simulink model "quadcopter_control_2018a"  (R2018a)
settings: Solver=VariableStepAuto  StartTime=0.0  StopTime=totTime  RelTol=1e-3
values from neighbouring files (symbols this model uses):
  armLength = 0.1    [quadcopter.m]    (also in quadcopter_control_RL.m)
  dragFactor = 0.1    [quadcopter.m]    (also in quadcopter_control_RL.m)
  iX = 0.03    [quadcopter.m]    (also in quadcopter_control_RL.m)
  iY = 0.03    [quadcopter.m]    (also in quadcopter_control_RL.m)
  iZ = 0.03    [quadcopter.m]    (also in quadcopter_control_RL.m)
  mass = 0.25    [quadcopter.m]    (also in quadcopter_control_RL.m)
  phi0 = 0.0    (= 0)    [quadcopter.m]    (also in quadcopter_control_RL.m = omega_vec_next(1))
  phiDot0 = 0.0    (= 0)    [quadcopter.m]    (also in quadcopter_control_RL.m = omega_vec_next(4))
  psi0 = 0.0    (= 0)    [quadcopter.m]    (also in quadcopter_control_RL.m = omega_vec_next(3))
  psiDot0 = 0.0    (= 0)    [quadcopter.m]    (also in quadcopter_control_RL.m = omega_vec_next(6))
  theta0 = 0.0    (= 0)    [quadcopter.m]    (also in quadcopter_control_RL.m = omega_vec_next(2))
  thetaDot0 = 0.0    (= 0)    [quadcopter.m]    (also in quadcopter_control_RL.m = omega_vec_next(5))
  thrustFactor = 0.1    [quadcopter.m]    (also in quadcopter_control_RL.m)
  trajectory = zeros(length(t),4)    [quadcopter.m]
  Ts = 0.1    [quadcopter.m]
  x0 = 0.0    (= 0)    [quadcopter.m]    (also in quadcopter_control_RL.m = x_vec_next(1))
  xDot0 = 0.0    (= 0)    [quadcopter.m]    (also in quadcopter_control_RL.m = x_vec_next(4))
  y0 = 0.0    (= 0)    [quadcopter.m]    (also in quadcopter_control_RL.m = x_vec_next(2))
  yDot0 = 0.0    (= 0)    [quadcopter.m]    (also in quadcopter_control_RL.m = x_vec_next(5))
  z0 = 0.00000001    (= 1e-08)    [quadcopter.m]    (also in quadcopter_control_RL.m = x_vec_next(3))
  zDot0 = 0.00000001    (= 1e-08)    [quadcopter.m]    (also in quadcopter_control_RL.m = x_vec_next(6))
libraries: simulink x1
settings Model: Creator=Ramprasad  LastModifiedBy=vickneshbalabaskara
settings DebuggingCC: LibraryContextMissingDiagnostic=warning
settings SFSimCC: SimUseLocalCustomCode=on
settings RTWCC: RTWUseLocalCustomCode=on

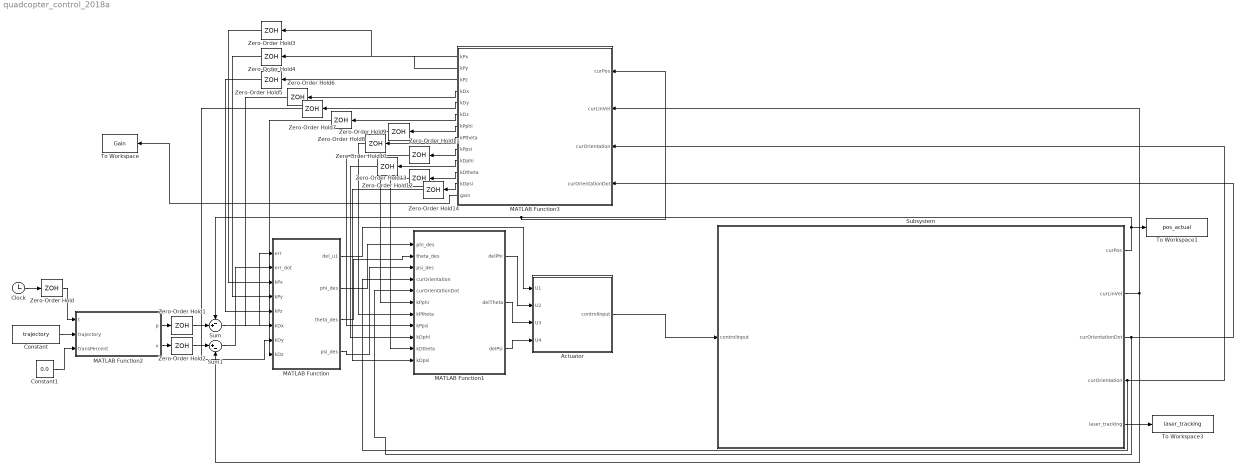
== system quadcopter_control_2018a ==
  Actuator : Subsystem
  Clock : Clock
  Constant : Constant  Value=trajectory
  Constant1 : Constant  Value=0.0
  MATLAB Function : MATLAB Function  TreatAsAtomicUnit=on
  MATLAB Function1 : MATLAB Function  TreatAsAtomicUnit=on
  MATLAB Function2 : MATLAB Function  TreatAsAtomicUnit=on
  MATLAB Function3 : MATLAB Function  TreatAsAtomicUnit=on
  Subsystem : Subsystem
  Sum : Sum  Inputs=-+|
  Sum1 : Sum  Inputs=|+-
  To Workspace : ToWorkspace  VariableName=Gain  SaveFormat=Timeseries  SampleTime=Ts
  To Workspace1 : ToWorkspace  VariableName=pos_actual  SaveFormat=Structure With Time  SampleTime=-1
  To Workspace3 : ToWorkspace  VariableName=laser_tracking  SaveFormat=Structure With Time  SampleTime=-1
  Zero-Order Hold{,1..14} (15 alike) : ZeroOrderHold  SampleTime=0.001
  wires:
  Actuator/1(controlInput) -> Subsystem/1(controlInput)
  Constant/1 -> MATLAB Function2/2(trajectory)
  Clock/1 -> Zero-Order Hold/1
  Zero-Order Hold/1 -> MATLAB Function2/1(t)
  MATLAB Function/2(phi_des) -> MATLAB Function1/1(phi_des)
  MATLAB Function/3(theta_des) -> MATLAB Function1/2(theta_des)
  MATLAB Function/4(psi_des) -> MATLAB Function1/3(psi_des)
  MATLAB Function2/1(p) -> Zero-Order Hold1/1
  MATLAB Function2/2(v) -> Zero-Order Hold2/1
  Zero-Order Hold1/1 -> Sum/2
  Zero-Order Hold2/1 -> Sum1/1
  Sum/1 -> MATLAB Function/1(err)
  Sum1/1 -> MATLAB Function/2(err_dot)
  Subsystem/1(curPos) -> MATLAB Function3/1(curPos), Sum/1, To Workspace1/1
  Constant1/1 -> MATLAB Function2/3(transPercent)
  MATLAB Function/1(del_u1) -> Actuator/1(U1)
  MATLAB Function1/1(delPhi) -> Actuator/2(U2)
  MATLAB Function1/2(delTheta) -> Actuator/3(U3)
  MATLAB Function1/3(delPsi) -> Actuator/4(U4)
  Subsystem/5(laser_tracking) -> To Workspace3/1
  Subsystem/2(curLinVel) -> Sum1/2, MATLAB Function3/2(curLinVel)
  Subsystem/4(curOrientation) -> MATLAB Function1/4(curOrientation), MATLAB Function3/3(curOrientation)
  Subsystem/3(curOrientationDot) -> MATLAB Function1/5(curOrientationDot), MATLAB Function3/4(curOrientationDot)
  MATLAB Function3/1(kPx) -> Zero-Order Hold3/1
  MATLAB Function3/2(kPy) -> Zero-Order Hold4/1
  MATLAB Function3/3(kPz) -> Zero-Order Hold5/1
  MATLAB Function3/4(kDx) -> Zero-Order Hold6/1
  MATLAB Function3/5(kDy) -> Zero-Order Hold7/1
  MATLAB Function3/6(kDz) -> Zero-Order Hold8/1
  MATLAB Function3/7(kPphi) -> Zero-Order Hold9/1
  MATLAB Function3/8(kPtheta) -> Zero-Order Hold10/1
  MATLAB Function3/9(kPpsi) -> Zero-Order Hold11/1
  MATLAB Function3/10(kDphi) -> Zero-Order Hold12/1
  MATLAB Function3/11(kDtheta) -> Zero-Order Hold13/1
  MATLAB Function3/12(kDpsi) -> Zero-Order Hold14/1
  Zero-Order Hold3/1 -> MATLAB Function/3(kPx)
  Zero-Order Hold4/1 -> MATLAB Function/4(kPy)
  Zero-Order Hold5/1 -> MATLAB Function/5(kPz)
  Zero-Order Hold6/1 -> MATLAB Function/6(kDx)
  Zero-Order Hold7/1 -> MATLAB Function/7(kDy)
  Zero-Order Hold8/1 -> MATLAB Function/8(kDz)
  Zero-Order Hold9/1 -> MATLAB Function1/6(kPphi)
  Zero-Order Hold10/1 -> MATLAB Function1/7(kPtheta)
  Zero-Order Hold11/1 -> MATLAB Function1/8(kPpsi)
  Zero-Order Hold12/1 -> MATLAB Function1/9(kDphi)
  Zero-Order Hold13/1 -> MATLAB Function1/10(kDtheta)
  Zero-Order Hold14/1 -> MATLAB Function1/11(kDpsi)
  MATLAB Function3/13(gain) -> To Workspace/1

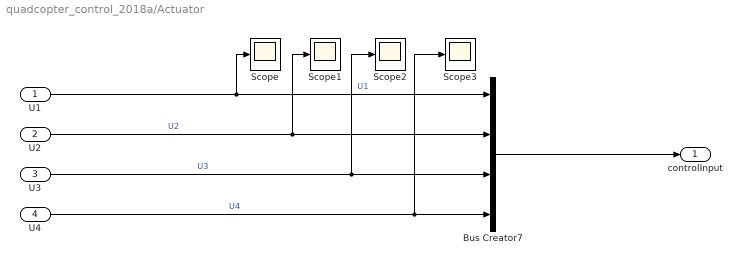
== system quadcopter_control_2018a/Actuator ==
  U1 : Inport
  U2 : Inport  Port=2
  U3 : Inport  Port=3
  U4 : Inport  Port=4
  Bus Creator7 : BusCreator  Inputs=4
  Scope{,1..3} (4 alike) : Scope
  controlInput : Outport
  wires:
  U1/1 -> Scope/1, Bus Creator7/1  "U1"
  U4/1 -> Scope3/1, Bus Creator7/4  "U4"
  Bus Creator7/1 -> controlInput/1
  U2/1 -> Scope1/1, Bus Creator7/2  "U2"
  U3/1 -> Scope2/1, Bus Creator7/3  "U3"

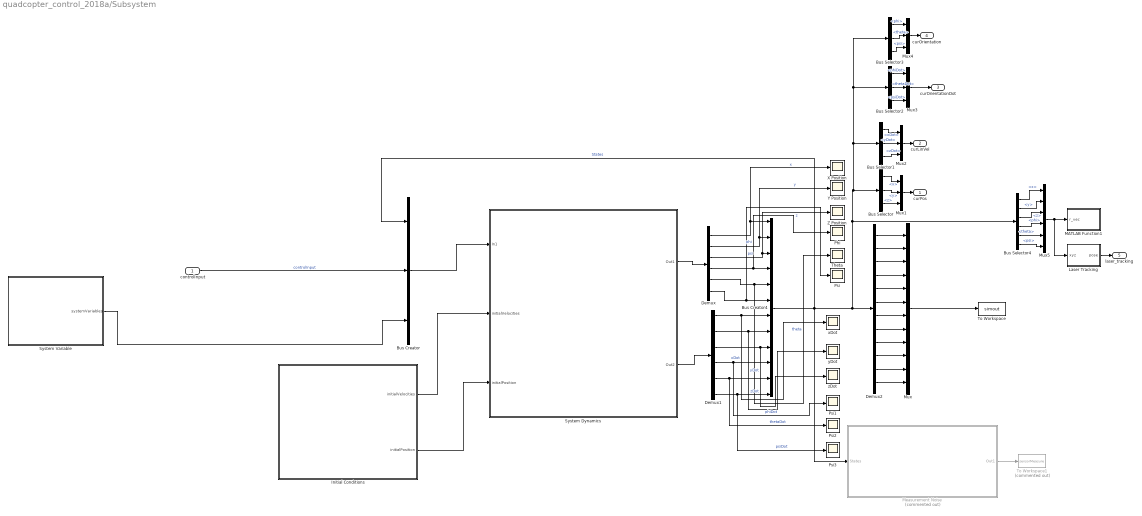
== system quadcopter_control_2018a/Subsystem ==
  controlInput : Inport
  Bus Creator : BusCreator  Inputs=3
  Bus Creator4 : BusCreator  Inputs=12
  Bus Selector : BusSelector  OutputSignals=x,y,z
  Bus Selector1 : BusSelector  OutputSignals=xDot,yDot,zDot
  Bus Selector2 : BusSelector  OutputSignals=phiDot,thetaDot,psiDot
  Bus Selector3 : BusSelector  OutputSignals=phi,theta,psi
  Bus Selector4 : BusSelector  OutputSignals=x,y,z,phi,theta,psi
  Demux : Demux  Outputs=6
  Demux1 : Demux  Outputs=6
  Demux2 : Demux  Outputs=12
  Initial Conditions : Subsystem
  Laser Tracking : MATLAB Function  TreatAsAtomicUnit=on
  MATLAB Function1 : MATLAB Function  TreatAsAtomicUnit=on
  Measurement Noise : Subsystem  Commented=on
  Mux : Mux  Inputs=12
  Mux{1..4} (4 alike) : Mux  Inputs=3
  Mux5 : Mux  Inputs=6
  Phi : Scope
  Psi{,1..3} (4 alike) : Scope
  System Dynamics : Subsystem
  System Variable : Subsystem
  Theta : Scope
  To Workspace : ToWorkspace  VariableName=simout  SaveFormat=Timeseries  SampleTime=Ts
  To Workspace1 : ToWorkspace  Commented=on  VariableName=sensorMeasure  SaveFormat=Timeseries  SampleTime=-1
  X Position : Scope
  Y Position : Scope
  Z Position : Scope
  xDot : Scope
  yDot : Scope
  zDot : Scope
  curPos : Outport
  curLinVel : Outport  Port=2
  curOrientationDot : Outport  Port=3
  curOrientation : Outport  Port=4
  laser_tracking : Outport  Port=5
  wires:
  Demux1/1 -> xDot/1, Bus Creator4/7  "xDot"
  Demux2/6 -> Mux/6
  Demux/6 -> Psi/1, Bus Creator4/6  "psi"
  Demux1/2 -> yDot/1, Bus Creator4/8  "yDot"
  Mux/1 -> To Workspace/1
  Demux2/9 -> Mux/9
  Demux1/6 -> Psi3/1, Bus Creator4/12  "psiDot"
  Measurement Noise/1(Out1) -> To Workspace1/1
  Demux/4 -> Phi/1, Bus Creator4/4  "phi"
  System Dynamics/1(Out1) -> Demux/1
  Initial Conditions/1(initialVelocities) -> System Dynamics/2(initialVelocities)
  Initial Conditions/2(initialPosition) -> System Dynamics/3(initialPosition)
  Bus Creator/1 -> System Dynamics/1(In1)
  Demux/2 -> Bus Creator4/2, Y Position/1  "y"
  Demux2/5 -> Mux/5
  System Dynamics/2(Out2) -> Demux1/1
  Demux2/3 -> Mux/3
  Demux/1 -> Bus Creator4/1, X Position/1  "x"
  Demux2/8 -> Mux/8
  Demux2/7 -> Mux/7
  Demux2/2 -> Mux/2
  Demux2/12 -> Mux/12
  Demux1/4 -> Psi1/1, Bus Creator4/10  "phiDot"
  Demux/5 -> Theta/1, Bus Creator4/5  "theta"
  Demux/3 -> Z Position/1, Bus Creator4/3  "z"
  Demux2/1 -> Mux/1
  Demux2/10 -> Mux/10
  Bus Creator4/1 -> Bus Creator/1, Bus Selector3/1, Bus Selector2/1, Bus Selector1/1, Bus Selector/1, Bus Selector4/1, Demux2/1, Measurement Noise/1(States)  "States"
  Demux2/11 -> Mux/11
  Demux1/5 -> Psi2/1, Bus Creator4/11  "thetaDot"
  Demux2/4 -> Mux/4
  Demux1/3 -> zDot/1, Bus Creator4/9  "zDot"
  System Variable/1(systemVariables) -> Bus Creator/3
  Bus Selector/3 -> Mux1/3  "<z>"
  Bus Selector/2 -> Mux1/2  "<y>"
  Bus Selector/1 -> Mux1/1  "<x>"
  Mux1/1 -> curPos/1
  Bus Selector1/2 -> Mux2/2  "<yDot>"
  Bus Selector1/3 -> Mux2/3  "<zDot>"
  Bus Selector1/1 -> Mux2/1  "<xDot>"
  Mux2/1 -> curLinVel/1
  Bus Selector3/1 -> Mux4/1  "<phi>"
  Bus Selector3/2 -> Mux4/2  "<theta>"
  Bus Selector3/3 -> Mux4/3  "<psi>"
  Mux4/1 -> curOrientation/1
  Bus Selector2/1 -> Mux3/1  "<phiDot>"
  Bus Selector2/2 -> Mux3/2  "<thetaDot>"
  Mux3/1 -> curOrientationDot/1
  Bus Selector2/3 -> Mux3/3  "<psiDot>"
  Bus Selector4/1 -> Mux5/1  "<x>"
  Bus Selector4/2 -> Mux5/2  "<y>"
  Bus Selector4/3 -> Mux5/3  "<z>"
  Bus Selector4/4 -> Mux5/4  "<phi>"
  Bus Selector4/5 -> Mux5/5  "<theta>"
  Bus Selector4/6 -> Mux5/6  "<psi>"
  Mux5/1 -> Laser Tracking/1(xyz), MATLAB Function1/1(r_vec)
  controlInput/1 -> Bus Creator/2  "controlInput"
  Laser Tracking/1(pose) -> laser_tracking/1

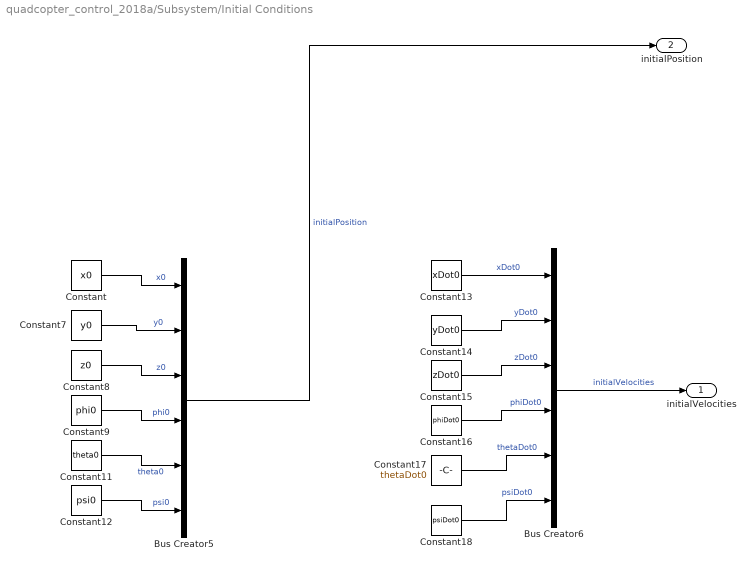
== system quadcopter_control_2018a/Subsystem/Initial Conditions ==
  Bus Creator5 : BusCreator  Inputs=6
  Bus Creator6 : BusCreator  Inputs=6
  Constant : Constant  Value=x0
  Constant11 : Constant  Value=theta0
  Constant12 : Constant  Value=psi0
  Constant13 : Constant  Value=xDot0
  Constant14 : Constant  Value=yDot0
  Constant15 : Constant  Value=zDot0
  Constant16 : Constant  Value=phiDot0
  Constant17 : Constant  Value=thetaDot0
  Constant18 : Constant  Value=psiDot0
  Constant7 : Constant  Value=y0
  Constant8 : Constant  Value=z0
  Constant9 : Constant  Value=phi0
  initialVelocities : Outport
  initialPosition : Outport  Port=2
  wires:
  Constant9/1 -> Bus Creator5/4  "phi0"
  Constant14/1 -> Bus Creator6/2  "yDot0"
  Constant17/1 -> Bus Creator6/5  "thetaDot0"
  Constant18/1 -> Bus Creator6/6  "psiDot0"
  Constant13/1 -> Bus Creator6/1  "xDot0"
  Constant11/1 -> Bus Creator5/5  "theta0"
  Constant8/1 -> Bus Creator5/3  "z0"
  Constant16/1 -> Bus Creator6/4  "phiDot0"
  Constant12/1 -> Bus Creator5/6  "psi0"
  Constant15/1 -> Bus Creator6/3  "zDot0"
  Constant/1 -> Bus Creator5/1  "x0"
  Bus Creator6/1 -> initialVelocities/1  "initialVelocities"
  Constant7/1 -> Bus Creator5/2  "y0"
  Bus Creator5/1 -> initialPosition/1  "initialPosition"

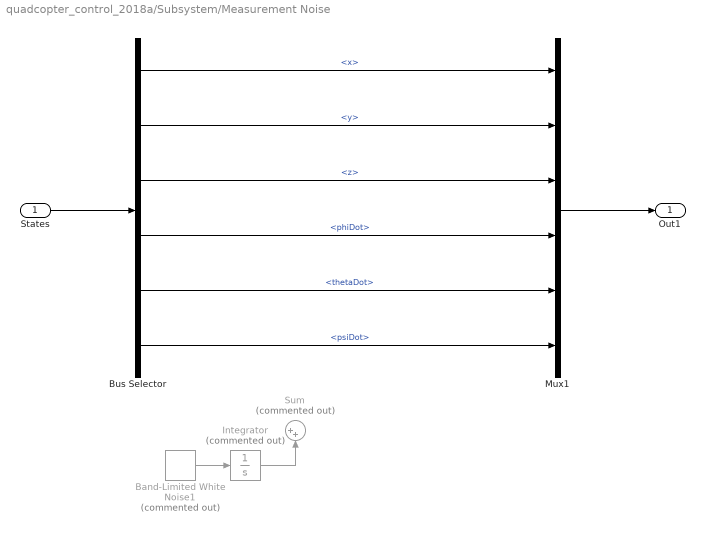
== system quadcopter_control_2018a/Subsystem/Measurement Noise ==
  States : Inport
  Band-Limited White Noise1 : simulink/Sources/Band-Limited White Noise  Commented=on  Cov=[0.0]  Ts=Ts  seed=[23341]
  Bus Selector : BusSelector  OutputSignals=x,y,z,phiDot,thetaDot,psiDot
  Integrator : Integrator  Commented=on
  Mux1 : Mux  Inputs=6
  Sum : Sum  Commented=on  Inputs=|++
  Out1 : Outport
  wires:
  Integrator/1 -> Sum/2
  Bus Selector/3 -> Mux1/3  "<z>"
  Bus Selector/2 -> Mux1/2  "<y>"
  Mux1/1 -> Out1/1
  Band-Limited White Noise1/1 -> Integrator/1
  Bus Selector/4 -> Mux1/4  "<phiDot>"
  States/1 -> Bus Selector/1
  Bus Selector/6 -> Mux1/6  "<psiDot>"
  Bus Selector/5 -> Mux1/5  "<thetaDot>"
  Bus Selector/1 -> Mux1/1  "<x>"

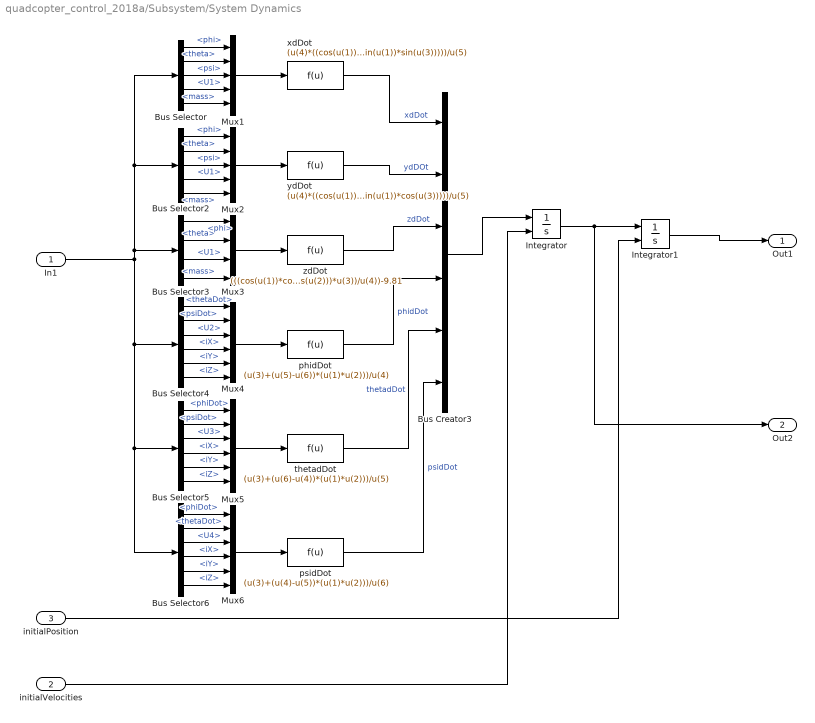
== system quadcopter_control_2018a/Subsystem/System Dynamics ==
  In1 : Inport
  initialVelocities : Inport  Port=2
  initialPosition : Inport  Port=3
  Bus Creator3 : BusCreator  Inputs=6
  Bus Selector : BusSelector  OutputSignals=States.phi,States.theta,States.psi,controlInput.U1,systemVariables.mass
  Bus Selector2 : BusSelector  OutputSignals=States.phi,States.theta,States.psi,controlInput.U1,systemVariables.mass
  Bus Selector3 : BusSelector  OutputSignals=States.phi,States.theta,controlInput.U1,systemVariables.mass
  Bus Selector4 : BusSelector  OutputSignals=States.thetaDot,States.psiDot,controlInput.U2,systemVariables.iX,systemVariables.iY,systemVariables.iZ
  Bus Selector5 : BusSelector  OutputSignals=States.phiDot,States.psiDot,controlInput.U3,systemVariables.iX,systemVariables.iY,systemVariables.iZ
  Bus Selector6 : BusSelector  OutputSignals=States.phiDot,States.thetaDot,controlInput.U4,systemVariables.iX,systemVariables.iY,systemVariables.iZ
  Integrator : Integrator  InitialConditionSource=external
  Integrator1 : Integrator  InitialConditionSource=external
  Mux1 : Mux  Inputs=5
  Mux2 : Mux  Inputs=5
  Mux3 : Mux
  Mux4 : Mux  Inputs=6
  Mux5 : Mux  Inputs=6
  Mux6 : Mux  Inputs=6
  phidDot : Fcn  Expr=(u(3)+(u(5)-u(6))*(u(1)*u(2)))/u(4)
  psidDot : Fcn  Expr=(u(3)+(u(4)-u(5))*(u(1)*u(2)))/u(6)
  thetadDot : Fcn  Expr=(u(3)+(u(6)-u(4))*(u(1)*u(2)))/u(5)
  xdDot : Fcn  Expr=(u(4)*((cos(u(1))*sin(u(2))*cos(u(3)))+(sin(u(1))*sin(u(3)))))/u(5)
  ydDot : Fcn  Expr=(u(4)*((cos(u(1))*sin(u(2))*sin(u(3)))-(sin(u(1))*cos(u(3)))))/u(5)
  zdDot : Fcn  Expr=(((cos(u(1))*cos(u(2)))*u(3))/u(4))-9.81
  Out1 : Outport
  Out2 : Outport  Port=2
  wires:
  initialPosition/1 -> Integrator1/2
  xdDot/1 -> Bus Creator3/1  "xdDot"
  Bus Selector2/2 -> Mux2/2  "<theta>"
  Bus Selector4/5 -> Mux4/5  "<iY>"
  Bus Selector2/4 -> Mux2/4  "<U1>"
  Bus Selector4/3 -> Mux4/3  "<U2>"
  thetadDot/1 -> Bus Creator3/5  "thetadDot"
  Bus Selector5/2 -> Mux5/2  "<psiDot>"
  Bus Selector2/1 -> Mux2/1  "<phi>"
  Mux5/1 -> thetadDot/1
  Bus Selector6/4 -> Mux6/4  "<iX>"
  Bus Selector5/6 -> Mux5/6  "<iZ>"
  Bus Selector6/2 -> Mux6/2  "<thetaDot>"
  phidDot/1 -> Bus Creator3/4  "phidDot"
  Bus Selector2/3 -> Mux2/3  "<psi>"
  In1/1 -> Bus Selector4/1, Bus Selector5/1, Bus Selector6/1, Bus Selector3/1, Bus Selector2/1, Bus Selector/1
  Bus Selector5/3 -> Mux5/3  "<U3>"
  Bus Selector3/2 -> Mux3/2  "<theta>"
  Bus Selector3/1 -> Mux3/1  "<phi>"
  initialVelocities/1 -> Integrator/2
  Bus Selector/3 -> Mux1/3  "<psi>"
  Mux6/1 -> psidDot/1
  Bus Selector5/4 -> Mux5/4  "<iX>"
  Bus Selector/4 -> Mux1/4  "<U1>"
  Bus Selector/1 -> Mux1/1  "<phi>"
  Mux4/1 -> phidDot/1
  Bus Selector4/6 -> Mux4/6  "<iZ>"
  Bus Selector2/5 -> Mux2/5  "<mass>"
  Bus Creator3/1 -> Integrator/1
  Bus Selector6/6 -> Mux6/6  "<iZ>"
  Bus Selector3/3 -> Mux3/3  "<U1>"
  Mux2/1 -> ydDot/1
  Bus Selector6/3 -> Mux6/3  "<U4>"
  Bus Selector6/1 -> Mux6/1  "<phiDot>"
  zdDot/1 -> Bus Creator3/3  "zdDot"
  Bus Selector5/1 -> Mux5/1  "<phiDot>"
  Bus Selector4/2 -> Mux4/2  "<psiDot>"
  Bus Selector6/5 -> Mux6/5  "<iY>"
  Bus Selector4/4 -> Mux4/4  "<iX>"
  Bus Selector4/1 -> Mux4/1  "<thetaDot>"
  Mux3/1 -> zdDot/1
  Integrator/1 -> Integrator1/1, Out2/1
  psidDot/1 -> Bus Creator3/6  "psidDot"
  Integrator1/1 -> Out1/1
  Bus Selector/5 -> Mux1/5  "<mass>"
  ydDot/1 -> Bus Creator3/2  "ydDOt"
  Bus Selector5/5 -> Mux5/5  "<iY>"
  Bus Selector/2 -> Mux1/2  "<theta>"
  Bus Selector3/4 -> Mux3/4  "<mass>"
  Mux1/1 -> xdDot/1

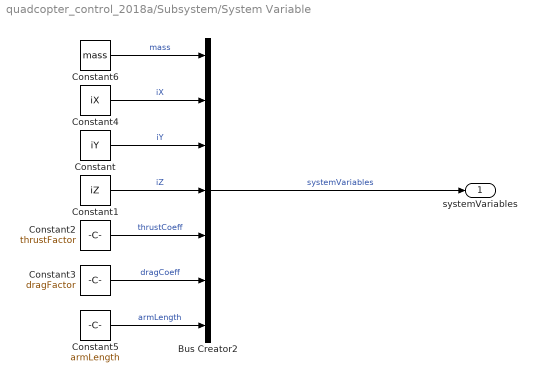
== system quadcopter_control_2018a/Subsystem/System Variable ==
  Bus Creator2 : BusCreator  Inputs=7
  Constant : Constant  Value=iY
  Constant1 : Constant  Value=iZ
  Constant2 : Constant  Value=thrustFactor
  Constant3 : Constant  Value=dragFactor
  Constant4 : Constant  Value=iX
  Constant5 : Constant  Value=armLength
  Constant6 : Constant  Value=mass
  systemVariables : Outport
  wires:
  Constant6/1 -> Bus Creator2/1  "mass"
  Constant2/1 -> Bus Creator2/5  "thrustCoeff"
  Constant/1 -> Bus Creator2/3  "iY"
  Constant1/1 -> Bus Creator2/4  "iZ"
  Constant3/1 -> Bus Creator2/6  "dragCoeff"
  Constant4/1 -> Bus Creator2/2  "iX"
  Constant5/1 -> Bus Creator2/7  "armLength"
  Bus Creator2/1 -> systemVariables/1  "systemVariables"

== matlab function quadcopter_control_2018a/Subsystem/MATLAB Function1 ==
  settings: updateMethod=DISCRETE
  data: r_vec input
function drawDrone(r_vec)
%#codegen
coder.extrinsic('evalin');
coder.extrinsic('load');
coder.extrinsic('animatedline');
% persistent figNum axisHandel Sim_Exact points3D;

% if isempty(Sim_Exact)
%     Sim_Exact = evalin('base','Sim_Exact');
%     a.points3D = zeros(21,3,'double');
%     a = load('points3D.mat');
%     points3D = zeros(21,3,'double');
%     points3D = a.points3D;
% end

x = r_vec(1);
y = r_vec(2);
z = r_vec(3);
phi = r_vec(4);
theta = r_vec(5);
psi = r_vec(6);

T06 = [cos(psi)*cos(theta) (cos(psi)*sin(theta)*sin(phi))-(sin(psi)*cos(phi)) (cos(phi)*sin(theta)*cos(psi))+(sin(phi)*sin(psi)) x;...
       sin(psi)*cos(theta) (sin(phi)*sin(theta)*sin(psi))+(cos(phi)*cos(psi)) (sin(psi)*sin(theta)*cos(phi))-(cos(psi)*sin(phi)) y;...
       -sin(theta) (cos(theta)*sin(phi)) (cos(theta)*cos(phi)) z;...
       0 0 0 1];

R06 = T06(1:3,1:3);

% P1 =[ 0
%     0
%     0.29];
% P2 = [ 0.27*cos(x)*cos(y);
%     0.27*cos(y)*sin(x);
%     0.29 - 0.27*sin(y)];
% P3 = [ 0.27*cos(x)*cos(y) - 0.07*cos(x)*sin(y)*sin(z) + 0.07*cos(x)*cos(y)*cos(z);
%     0.27*cos(y)*sin(x) - 0.07*sin(x)*sin(y)*sin(z) + 0.07*cos(y)*cos(z)*sin(x);
%     0.29 - 0.07*cos(y)*sin(z) - 0.07*cos(z)*sin(y) - 0.27*sin(y)];
% 
% P4 = [ 0.27*cos(x)*cos(y) - 0.07*cos(x)*sin(y)*sin(z) + 0.07*cos(x)*cos(y)*cos(z) - 0.302*cos(x)*cos(y)*sin(z) - 0.302*cos(x)*cos(z)*sin(y);
%     0.27*cos(y)*sin(x) - 0.302*cos(y)*sin(x)*sin(z) - 0.302*cos(z)*sin(x)*sin(y) - 0.07*sin(x)*sin(y)*sin(z) + 0.07*cos(y)*cos(z)*sin(x);
%     0.302*sin(y)*sin(z) - 0.302*cos(y)*cos(z) - 0.07*cos(y)*sin(z) - 0.07*cos(z)*sin(y) - 0.27*sin(y) + 0.29];
% P5 = [ 0.27*cos(x)*cos(y) - 0.07*cos(x)*sin(y)*sin(z) + 0.07*cos(x)*cos(y)*cos(z) - 0.302*cos(x)*cos(y)*sin(z) - 0.302*cos(x)*cos(z)*sin(y)
%     0.27*cos(y)*sin(x) - 0.302*cos(y)*sin(x)*sin(z) - 0.302*cos(z)*sin(x)*sin(y) - 0.07*sin(x)*sin(y)*sin(z) + 0.07*cos(y)*cos(z)*sin(x)
%     0.302*sin(y)*sin(z) - 0.302*cos(y)*cos(z) - 0.07*cos(y)*sin(z) - 0.07*cos(z)*sin(y) - 0.27*sin(y) + 0.29];
% 
% P6 =[ 0.27*cos(x)*cos(y) - 0.07*cos(x)*sin(y)*sin(z) - 0.072*sin(x)*sin(phi)*sin(theta) + 0.07*cos(x)*cos(y)*cos(z) - 0.302*cos(x)*cos(y)*sin(z) - 0.302*cos(x)*cos(z)*sin(y) - 0.072*cos(x)*cos(y)*cos(theta)*sin(z) - 0.072*cos(x)*cos(z)*cos(theta)*sin(y) - 0.072*cos(x)*cos(y)*cos(z)*cos(phi)*sin(theta) + 0.072*cos(x)*cos(phi)*sin(y)*sin(z)*sin(theta);
%     0.27*cos(y)*sin(x) - 0.302*cos(y)*sin(x)*sin(z) - 0.302*cos(z)*sin(x)*sin(y) + 0.072*cos(x)*sin(phi)*sin(theta) - 0.07*sin(x)*sin(y)*sin(z) + 0.07*cos(y)*cos(z)*sin(x) - 0.072*cos(y)*cos(theta)*sin(x)*sin(z) - 0.072*cos(z)*cos(theta)*sin(x)*sin(y) - 0.072*cos(y)*cos(z)*cos(phi)*sin(x)*sin(theta) + 0.072*cos(phi)*sin(x)*sin(y)*sin(z)*sin(theta);
%     0.302*sin(y)*sin(z) - 0.302*cos(y)*cos(z) - 0.07*cos(y)*sin(z) - 0.07*cos(z)*sin(y) - 0.27*sin(y) + 0.072*cos(theta)*sin(y)*sin(z) - 0.072*cos(y)*cos(z)*cos(theta) + 0.072*cos(y)*cos(phi)*sin(z)*sin(theta) + 0.072*cos(z)*cos(phi)*sin(y)*sin(theta) + 0.29];

Q1 = [(0.1/sqrt(2));(0.1/sqrt(2));0];
Q2 = [-(0.1/sqrt(2));(0.1/sqrt(2));0];
Q3 = [(0.1/sqrt(2));-(0.1/sqrt(2));0];
Q4 = [-(0.1/sqrt(2));-(0.1/sqrt(2));0];

R1 = R06*Q1;
R2 = R06*Q2;
R3 = R06*Q3;
R4 = R06*Q4;

P1 = [x+R1(1);y+R1(2);z+R1(3)];
P2 = [x+R2(1);y+R2(2);z+R2(3)];
P3 = [x+R3(1);y+R3(2);z+R3(3)];
P4 = [x+R4(1);y+R4(2);z+R4(3)];

% if isempty(figNum)
%     figNum = figure(1);
%     hold on;
%     plot3([0;P1(1);P2(1);P3(1);P4(1);P5(1);P6(1)],...
%         [0;P1(2);P2(2);P3(2);P4(2);P5(2);P6(2)],...
%         [0;P1(3);P2(3);P3(3);P4(3);P5(3);P6(3)],'k','linewidth',2);
%     axisHandel = gca;
%     plot3([P6(1);P6(1)+T06(1,1)*.1],...
%         [P6(2);P6(2)+T06(2,1)*.1],...
%         [P6(3);P6(3)+T06(3,1)*.1],'r','Parent',axisHandel);
%     plot3([P6(1);P6(1)+T06(1,2)*.1],...
%         [P6(2);P6(2)+T06(2,2)*.1],...
%         [P6(3);P6(3)+T06(3,2)*.1],'g','Parent',axisHandel);
%     plot3([P6(1);P6(1)+T06(1,3)*.1],...
%         [P6(2);P6(2)+T06(2,3)*.1],...
%         [P6(3);P6(3)+T06(3,3)*.1],'b','Parent',axisHandel);
%     plot3(points3D(:,1),points3D(:,2),points3D(:,3),'m','Parent',axisHandel);
%     hold off;
%     axis([-.75 .75 -.75 .75 -.4 .75]);
%     axisHandel = gca;
% else
figure(1)
plot3([x;P1(1)],[y;P1(2)],[z;P1(3)],'k','linewidth',2,'Parent',gca);
hold on;
plot3([x;P2(1)],[y;P2(2)],[z;P2(3)],'k','linewidth',2,'Parent',gca);
hold on;
plot3([x;P3(1)],[y;P3(2)],[z;P3(3)],'k','linewidth',2,'Parent',gca);
hold on;
plot3([x;P4(1)],[y;P4(2)],[z;P4(3)],'k','linewidth',2,'Parent',gca);
hold on;
plot3([x;x+T06(1,1)*.1],[y;y+T06(2,1)*.1],[z;z+T06(3,1)*.1],'r','Parent',gca);
plot3([x;x+T06(1,2)*.1],[y;y+T06(2,2)*.1],[z;z+T06(3,2)*.1],'g','Parent',gca);
plot3([x;x+T06(1,3)*.1],[y;y+T06(2,3)*.1],[z;z+T06(3,3)*.1],'b','Parent',gca);
% plot3([P6(1);P6(1)+T06(1,2)*.1],...
%     [P6(2);P6(2)+T06(2,2)*.1],...
%     [P6(3);P6(3)+T06(3,2)*.1],'g','Parent',gca);
% plot3([P6(1);P6(1)+T06(1,3)*.1],...
%     [P6(2);P6(2)+T06(2,3)*.1],...
%     [P6(3);P6(3)+T06(3,3)*.1],'b','Parent',gca);
% plot3(x,y,z,'m','Parent',gca);
hold off;
axis([-0.1 1.1 -0.1 1.1 0.0 1.1]);
end

== matlab function quadcopter_control_2018a/MATLAB Function2 ==
  data: t input; p output; trajectory input; transPercent input; v output
function [p,v] = constAccelInterp(t,trajectory,transPercent)
pTime = trajectory(:,1);
[n,m] = size(trajectory);
p = zeros(1,m-1);
v = zeros(1,m-1);
a = zeros(1,m-1);
for j = 2:n-1
    if j-1==1 && t>pTime(j-1,1) && t<(pTime(j-1,1)+transPercent)
        for i = 2:m
            p(1,i-1) = trajectory(j-1,i) +...
                (((trajectory(j,i)-trajectory(j-1,i))*((t-pTime(j-1,1)+transPercent)^2))/(4*transPercent*(pTime(j,1)-pTime(j-1,1))));
            v(1,i-1) = (((trajectory(j,i)-trajectory(j-1,i))*(t-pTime(j-1,1)+transPercent))/(2*transPercent*(pTime(j,1)-pTime(j-1,1))));
            a(1,i-1) = ((trajectory(j,i)-trajectory(j-1,i))/(2*transPercent*(pTime(j,1)-pTime(j-1,1))));
        end
        break;
    elseif j+1==n && t>(pTime(j+1,1)-transPercent) && t<pTime(j+1,1)
        for i = 2:m
            p(1,i-1) = trajectory(j+1,i) - ...
                (((trajectory(j+1,i)-trajectory(j,i))*((t-pTime(j+1,1)-transPercent)^2))/(4*transPercent*(pTime(j+1,1)-pTime(j,1))));
            v(1,i-1) = -(((trajectory(j+1,i)-trajectory(j,i))*(t-pTime(j+1,1)-transPercent))/(2*transPercent*(pTime(j+1,1)-pTime(j,1))));
            a(1,i-1) = -((trajectory(j+1,i)-trajectory(j,i))/(2*transPercent*(pTime(j+1,1)-pTime(j,1))));
        end
        break;
    elseif t>(pTime(j-1,1)+transPercent) && t<(pTime(j,1)-transPercent)
        for i = 2:m
            p(1,i-1) = trajectory(j,i)-(((pTime(j,1)-t)*(trajectory(j,i)-...
                trajectory(j-1,i)))/(pTime(j,1)-pTime(j-1,1)));
            v(1,i-1) = (trajectory(j,i)-trajectory(j-1,i))/(pTime(j,1)-pTime(j-1,1));
            a(1,i-1) = 0.0;
        end
        break;
    elseif t>(pTime(j,1)-transPercent) && t<(pTime(j,1)+transPercent)
        for i = 2:m
            p(1,i-1) = trajectory(j,i) - ...
                (((trajectory(j,i)-trajectory(j-1,i))*((t-pTime(j,1)-transPercent)^2))/(4*transPercent*(pTime(j,1)-pTime(j-1,1)))) +...
                (((trajectory(j+1,i)-trajectory(j,i))*((t-pTime(j,1)+transPercent)^2))/(4*transPercent*(pTime(j+1,1)-pTime(j,1))));
            v(1,i-1) = -(((trajectory(j,i)-trajectory(j-1,i))*(t-pTime(j,1)-transPercent))/(2*transPercent*(pTime(j,1)-pTime(j-1,1)))) +...
                (((trajectory(j+1,i)-trajectory(j,i))*(t-pTime(j,1)+transPercent))/(2*transPercent*(pTime(j+1,1)-pTime(j,1))));
            a(1,i-1) = -((trajectory(j,i)-trajectory(j-1,i))/(2*transPercent*(pTime(j,1)-pTime(j-1,1)))) + ...
                ((trajectory(j+1,i)-trajectory(j,i))/(2*transPercent*(pTime(j+1,1)-pTime(j,1))));
        end
        break;
    elseif t>(pTime(j,1)+transPercent) && t<(pTime(j+1,1)-transPercent)
        for i = 2:m
            p(1,i-1) = trajectory(j,i)+(((t-pTime(j,1))*(trajectory(j+1,i)-...
                trajectory(j,i)))/(pTime(j+1,1)-pTime(j,1)));
            v(1,i-1) = (trajectory(j+1,i)-trajectory(j,i))/(pTime(j+1,1)-pTime(j,1));
            a(1,i-1) = 0.0;
        end    
        break;
    end
end
end

== matlab function quadcopter_control_2018a/MATLAB Function ==
  data: err input; err_dot input; del_u1 output; phi_des output; theta_des output; psi_des output; kPx input; kPy input; kPz input; kDx input; kDy input; kDz input
function [del_u1,phi_des,theta_des,psi_des] = POS_contol( err, err_dot, kPx,kPy,kPz,kDx,kDy,kDz)
%

% Q1 = Q(:,:,1);
% Q2 = Q(:,:,2);
% Q3 = Q(:,:,3);
% Q4 = Q(:,:,4);
% Q5 = Q(:,:,5);
% Q6 = Q(:,:,6);

% Q7 = Q(:,:,7);
% Q8 = Q(:,:,8);
% Q9 = Q(:,:,9);
% Q10 = Q(:,:,10);
% Q11 = Q(:,:,11);
% Q12 = Q(:,:,12);

% kPz = 20.0;
% kDz = 20.0;
% kPx = 10.0;
% kDx = 20.0;
% kPy = 10.0;
% kDy = 20.0;
% 
% kPx_vec = kP(:,1);
% kPy_vec = kP(:,2);
% kPz_vec = kP(:,3);
% 
% kDx_vec = kD(:,1);
% kDy_vec = kD(:,2);
% kDz_vec = kD(:,3);
% for count = 0:25
%     if (t >= 0.1*count) && (t < 0.1*(count+1))
%         [~,I1] = max(Q1(count+1,:));
%         kPx = kPx_vec(I1);
%         [~,I2] = max(Q2(count+1,:));
%         kPy = kPy_vec(I2);
%         [~,I3] = max(Q3(count+1,:));
%         kPz = kPz_vec(I3);
% %         [~,I4] = max(Q5(count+1,:));
% %         kPphi = kPx_vec(I4);
% %         [~,I5] = max(Q6(count+1,:));
% %         kPtheta = kPx_vec(I5);
% %         [~,I6] = max(Q1(count+1,:));
% %         kPpsi = kPx_vec(I6);
%         [~,I7] = max(Q7(count+1,:));
%         kDx = kDx_vec(I7);
%         [~,I8] = max(Q8(count+1,:));
%         kDy = kDy_vec(I8);
%         [~,I9] = max(Q9(count+1,:));
%         kDz = kDz_vec(I9);
% %         [~,I10] = max(Q10(count+1,:));
% %         kDphi = kDx_vec(I10);
% %         [~,I11] = max(Q11(count+1,:));
% %         kDtheta = kDx_vec(I11);
% %         [~,I12] = max(Q12(count+1,:));
% %         kDpsi = kDx_vec(I12);
%     end
% end
psiDes = 0.0;
%
delOmegaH = sqrt((0.25*9.81)/(4*0.1));
%
zerr = err(3);
zerr_dot = err_dot(3);
z_ddot = kPz*(zerr) + kDz*zerr_dot + (0.25*9.81);
%
xerr = err(1);
xerr_dot = err_dot(1);
x_ddot = kPx*xerr + kDx*xerr_dot;
yerr = err(2);
yerr_dot = err_dot(2);
y_ddot = kPy*yerr + kDy*yerr_dot;
%
del_u1 = 0.9*z_ddot;
psi_des = psiDes;
%phi_des = ((rx_ddot*tan(psiDes) - ry_ddot)/rz_ddot)/(tan(psiDes)*sin(psiDes)+cos(psiDes));
%theta_des = ((rx_ddot/rz_ddot) - phi_des*sin(psiDes))/cos(psiDes);
%phi_des = (rx_ddot*sin(psiDes) - ry_ddot*cos(psiDes))/9.81;
%theta_des = (rx_ddot*cos(psiDes) + ry_ddot*sin(psiDes))/9.81;
R = [sin(psiDes) cos(psiDes);-cos(psiDes) sin(psiDes)];
invR = (0.25/del_u1)*inv(R);
%
phi_des = invR(1,:)*[x_ddot;y_ddot];
theta_des = invR(2,:)*[x_ddot;y_ddot];
%
end

== matlab function quadcopter_control_2018a/Subsystem/Laser Tracking ==
  data: xyz input; pose output
function pose = laserTracker(xyz)
%#codegen
coder.extrinsic('evalin');
% persistent Sim_Exact;
% 
% if isempty(Sim_Exact)
%     Sim_Exact = evalin('base','Sim_Exact');
% end


x = xyz(1,1);
y = xyz(2,1);
z = xyz(3,1);
    
% pose = [ sin(th6)*(cos(th4)*sin(th1) + sin(th4)*(cos(th1)*sin(th2)*sin(th3) - cos(th1)*cos(th2)*cos(th3))) + cos(th6)*(cos(th5)*(sin(th1)*sin(th4) - cos(th4)*(cos(th1)*sin(th2)*sin(th3) - cos(th1)*cos(th2)*cos(th3))) - sin(th5)*(cos(th1)*cos(th2)*sin(th3) + cos(th1)*cos(th3)*sin(th2))), cos(th6)*(cos(th4)*sin(th1) + sin(th4)*(cos(th1)*sin(th2)*sin(th3) - cos(th1)*cos(th2)*cos(th3))) - sin(th6)*(cos(th5)*(sin(th1)*sin(th4) - cos(th4)*(cos(th1)*sin(th2)*sin(th3) - cos(th1)*cos(th2)*cos(th3))) - sin(th5)*(cos(th1)*cos(th2)*sin(th3) + cos(th1)*cos(th3)*sin(th2))), - sin(th5)*(sin(th1)*sin(th4) - cos(th4)*(cos(th1)*sin(th2)*sin(th3) - cos(th1)*cos(th2)*cos(th3))) - cos(th5)*(cos(th1)*cos(th2)*sin(th3) + cos(th1)*cos(th3)*sin(th2)), (151838081588107*cos(th1)*cos(th2))/562949953421312 - (123928564092639*sin(th1))/72057594037927936 - (7184037743251309*cos(th1))/36893488147419103232 - (7330531551818703*cos(th4)*sin(th1))/36893488147419103232 - (5489399374888815*sin(th1)*sin(th4))/9223372036854775808 + (970893499285375*cos(th5)*(sin(th1)*sin(th4) - cos(th4)*(cos(th1)*sin(th2)*sin(th3) - cos(th1)*cos(th2)*cos(th3))))/9223372036854775808 - (5192391675427195*sin(th5)*(sin(th1)*sin(th4) - cos(th4)*(cos(th1)*sin(th2)*sin(th3) - cos(th1)*cos(th2)*cos(th3))))/72057594037927936 + (1663072680156839*sin(th6)*(cos(th4)*sin(th1) + sin(th4)*(cos(th1)*sin(th2)*sin(th3) - cos(th1)*cos(th2)*cos(th3))))/2305843009213693952 + (1663072680156839*cos(th6)*(cos(th5)*(sin(th1)*sin(th4) - cos(th4)*(cos(th1)*sin(th2)*sin(th3) - cos(th1)*cos(th2)*cos(th3))) - sin(th5)*(cos(th1)*cos(th2)*sin(th3) + cos(th1)*cos(th3)*sin(th2))))/2305843009213693952 + (5489399374888815*cos(th4)*(cos(th1)*sin(th2)*sin(th3) - cos(th1)*cos(th2)*cos(th3)))/9223372036854775808 - (5192391675427195*cos(th5)*(cos(th1)*cos(th2)*sin(th3) + cos(th1)*cos(th3)*sin(th2)))/72057594037927936 - (7330531551818703*sin(th4)*(cos(th1)*sin(th2)*sin(th3) - cos(th1)*cos(th2)*cos(th3)))/36893488147419103232 - (970893499285375*sin(th5)*(cos(th1)*cos(th2)*sin(th3) + cos(th1)*cos(th3)*sin(th2)))/9223372036854775808 - (1259578569946919*cos(th1)*sin(th2)*sin(th3))/18014398509481984 + (1259578569946919*cos(th1)*cos(th2)*cos(th3))/18014398509481984 - (5430591396830085*cos(th1)*cos(th2)*sin(th3))/18014398509481984 - (5430591396830085*cos(th1)*cos(th3)*sin(th2))/18014398509481984;
%     - sin(th6)*(cos(th1)*cos(th4) - sin(th4)*(sin(th1)*sin(th2)*sin(th3) - cos(th2)*cos(th3)*sin(th1))) - cos(th6)*(cos(th5)*(cos(th1)*sin(th4) + cos(th4)*(sin(th1)*sin(th2)*sin(th3) - cos(th2)*cos(th3)*sin(th1))) + sin(th5)*(cos(th2)*sin(th1)*sin(th3) + cos(th3)*sin(th1)*sin(th2))), sin(th6)*(cos(th5)*(cos(th1)*sin(th4) + cos(th4)*(sin(th1)*sin(th2)*sin(th3) - cos(th2)*cos(th3)*sin(th1))) + sin(th5)*(cos(th2)*sin(th1)*sin(th3) + cos(th3)*sin(th1)*sin(th2))) - cos(th6)*(cos(th1)*cos(th4) - sin(th4)*(sin(th1)*sin(th2)*sin(th3) - cos(th2)*cos(th3)*sin(th1))), sin(th5)*(cos(th1)*sin(th4) + cos(th4)*(sin(th1)*sin(th2)*sin(th3) - cos(th2)*cos(th3)*sin(th1))) - cos(th5)*(cos(th2)*sin(th1)*sin(th3) + cos(th3)*sin(th1)*sin(th2)), (123928564092639*cos(th1))/72057594037927936 - (7184037743251309*sin(th1))/36893488147419103232 + (7330531551818703*cos(th1)*cos(th4))/36893488147419103232 + (151838081588107*cos(th2)*sin(th1))/562949953421312 + (5489399374888815*cos(th1)*sin(th4))/9223372036854775808 - (970893499285375*cos(th5)*(cos(th1)*sin(th4) + cos(th4)*(sin(th1)*sin(th2)*sin(th3) - cos(th2)*cos(th3)*sin(th1))))/9223372036854775808 + (5192391675427195*sin(th5)*(cos(th1)*sin(th4) + cos(th4)*(sin(th1)*sin(th2)*sin(th3) - cos(th2)*cos(th3)*sin(th1))))/72057594037927936 - (1663072680156839*sin(th6)*(cos(th1)*cos(th4) - sin(th4)*(sin(th1)*sin(th2)*sin(th3) - cos(th2)*cos(th3)*sin(th1))))/2305843009213693952 + (5489399374888815*cos(th4)*(sin(th1)*sin(th2)*sin(th3) - cos(th2)*cos(th3)*sin(th1)))/9223372036854775808 - (5192391675427195*cos(th5)*(cos(th2)*sin(th1)*sin(th3) + cos(th3)*sin(th1)*sin(th2)))/72057594037927936 - (1663072680156839*cos(th6)*(cos(th5)*(cos(th1)*sin(th4) + cos(th4)*(sin(th1)*sin(th2)*sin(th3) - cos(th2)*cos(th3)*sin(th1))) + sin(th5)*(cos(th2)*sin(th1)*sin(th3) + cos(th3)*sin(th1)*sin(th2))))/2305843009213693952 - (7330531551818703*sin(th4)*(sin(th1)*sin(th2)*sin(th3) - cos(th2)*cos(th3)*sin(th1)))/36893488147419103232 - (970893499285375*sin(th5)*(cos(th2)*sin(th1)*sin(th3) + cos(th3)*sin(th1)*sin(th2)))/9223372036854775808 - (5430591396830085*cos(th2)*sin(th1)*sin(th3))/18014398509481984 - (5430591396830085*cos(th3)*sin(th1)*sin(th2))/18014398509481984 - (1259578569946919*sin(th1)*sin(th2)*sin(th3))/18014398509481984 + (1259578569946919*cos(th2)*cos(th3)*sin(th1))/18014398509481984;
%     sin(th4)*sin(th6)*(cos(th2)*sin(th3) + cos(th3)*sin(th2)) - cos(th6)*(sin(th5)*(cos(th2)*cos(th3) - sin(th2)*sin(th3)) + cos(th4)*cos(th5)*(cos(th2)*sin(th3) + cos(th3)*sin(th2))), sin(th6)*(sin(th5)*(cos(th2)*cos(th3) - sin(th2)*sin(th3)) + cos(th4)*cos(th5)*(cos(th2)*sin(th3) + cos(th3)*sin(th2))) + cos(th6)*sin(th4)*(cos(th2)*sin(th3) + cos(th3)*sin(th2)), cos(th4)*sin(th5)*(cos(th2)*sin(th3) + cos(th3)*sin(th2)) - cos(th5)*(cos(th2)*cos(th3) - sin(th2)*sin(th3)), (5430591396830085*sin(th2)*sin(th3))/18014398509481984 - (5430591396830085*cos(th2)*cos(th3))/18014398509481984 - (1259578569946919*cos(th2)*sin(th3))/18014398509481984 - (1259578569946919*cos(th3)*sin(th2))/18014398509481984 - (1663072680156839*cos(th6)*(sin(th5)*(cos(th2)*cos(th3) - sin(th2)*sin(th3)) + cos(th4)*cos(th5)*(cos(th2)*sin(th3) + cos(th3)*sin(th2))))/2305843009213693952 - (151838081588107*sin(th2))/562949953421312 + (5489399374888815*cos(th4)*(cos(th2)*sin(th3) + cos(th3)*sin(th2)))/9223372036854775808 - (5192391675427195*cos(th5)*(cos(th2)*cos(th3) - sin(th2)*sin(th3)))/72057594037927936 - (7330531551818703*sin(th4)*(cos(th2)*sin(th3) + cos(th3)*sin(th2)))/36893488147419103232 - (970893499285375*sin(th5)*(cos(th2)*cos(th3) - sin(th2)*sin(th3)))/9223372036854775808 - (970893499285375*cos(th4)*cos(th5)*(cos(th2)*sin(th3) + cos(th3)*sin(th2)))/9223372036854775808 + (5192391675427195*cos(th4)*sin(th5)*(cos(th2)*sin(th3) + cos(th3)*sin(th2)))/72057594037927936 + (1663072680156839*sin(th4)*sin(th6)*(cos(th2)*sin(th3) + cos(th3)*sin(th2)))/2305843009213693952 + 325695105792877/1125899906842624;
%     0, 0, 0, 1];

pose = [x;y;z];
end

== matlab function quadcopter_control_2018a/MATLAB Function1 ==
  data: phi_des input; theta_des input; psi_des input; curOrientation input; delPhi output; curOrientationDot input; delTheta output; delPsi output; kPphi input; kPtheta input; kPpsi input; kDphi input; kDtheta input; kDpsi input
function [delPhi, delTheta, delPsi] = Attitude_contol(phi_des,theta_des,psi_des,curOrientation,curOrientationDot,kPphi,kPtheta,kPpsi,kDphi,kDtheta,kDpsi)
%
% kPphi = 90.0;
% kDphi = 58.0;
% kPtheta = 95.0;
% kDtheta = 58.0;
% kPpsi = 20.0;
% kDpsi = 0.0;
%
delPhi = 0;
delTheta = 0;
delPsi = 0;
% Q4 = Q(:,:,4);
% Q5 = Q(:,:,5);
% Q6 = Q(:,:,6);
% 
% Q10 = Q(:,:,10);
% Q11 = Q(:,:,11);
% Q12 = Q(:,:,12);


% kPphi_vec = kP(:,1);
% kPtheta_vec = kP(:,2);
% kPpsi_vec = kP(:,3);
% 
% kDphi_vec = kD(:,1);
% kDtheta_vec = kD(:,2);
% kDpsi_vec = kD(:,3);
% for count = 0:25
%     if (t >= 0.1*count) && (t < 0.1*(count+1))
%         [~,I4] = max(Q4(count+1,:));
%         kPphi = kPphi_vec(I4);
%         [~,I5] = max(Q5(count+1,:));
%         kPtheta = kPtheta_vec(I5);
%         [~,I6] = max(Q6(count+1,:));
%         kPpsi = kPpsi_vec(I6);
%         [~,I10] = max(Q10(count+1,:));
%         kDphi = kDphi_vec(I10);
%         [~,I11] = max(Q11(count+1,:));
%         kDtheta = kDtheta_vec(I11);
%         [~,I12] = max(Q12(count+1,:));
%         kDpsi = kDpsi_vec(I12);
%     end
% end

err = [phi_des;theta_des;psi_des] - curOrientation;
errDot = -1*curOrientationDot;
%
delPhi = 0.9*(kPphi*err(1) + kDphi*errDot(1));
delTheta = 0.9*(kPtheta*err(2) + kDtheta*errDot(2));
delPsi = 0.9*(kPpsi*err(3) + kDpsi*errDot(3));
%
% delOmegaH = sqrt((0.25*9.81)/(4*0.1));
% %
% delOmegaVec = [delOmegaH+del_u1;delPhi;delTheta;delPsi];
% %
% R = [1 1 -1 1;...
%     1 1 1 -1;...
%     1 -1 1 1;...
%     1 -1 -1 -1];
% %
% omega1 = R(1,:)*delOmegaVec;
% omega2 = R(2,:)*delOmegaVec;
% omega3 = R(3,:)*delOmegaVec;
% omega4 = R(4,:)*delOmegaVec;
%
end

== matlab function quadcopter_control_2018a/MATLAB Function3 ==
  data: curPos input; curLinVel input; curOrientation input; kPx output; kPy output; kPz output; kDx output; curOrientationDot input; kDy output; kDz output; kPphi output; kPtheta output; kPpsi output; kDphi output; kDtheta output; kDpsi output; gain output
function [kPx,kPy,kPz,kDx,kDy,kDz,kPphi,kPtheta,kPpsi,kDphi,kDtheta,kDpsi,gain] = Discritization(curPos,curLinVel,curOrientation,curOrientationDot)
%
Q_file = load('Q_matrices.mat','Q');
kP_file = load('kP_vectors.mat','kP');
kD_file = load('kD_vectors.mat','kD');
gain = zeros(12,1);
Q = Q_file.Q(:,:,:);
kP = kP_file.kP(:,:);
kD = kD_file.kD(:,:);

kPx = 0;
kPy = 0;
kPz = 0;
kPphi = 0;
kPtheta = 0;
kPpsi = 0;

kDx = 0;
kDy = 0;
kDz = 0;
kDphi = 0;
kDtheta = 0;
kDpsi = 0;

N=26;

X_min = zeros(3,1);
X_max = ones(3,1);
%
omega_min = -0.3*ones(3,1);
omega_max = 0.3*ones(3,1);
%
X_dot_min = zeros(3,1);
X_dot_max = ones(3,1);
%
omega_dot_min = -1.5* ones(3,1);
omega_dot_max = 1.5 * ones(3,1);

Q_1 = Q(:,:,1);
Q_2 = Q(:,:,2);
Q_3 = Q(:,:,3);
Q_4 = Q(:,:,4);
Q_5 = Q(:,:,5);
Q_6 = Q(:,:,6);
Q_7 = Q(:,:,7);
Q_8 = Q(:,:,8);
Q_9 = Q(:,:,9);
Q_10 = Q(:,:,10);
Q_11 = Q(:,:,11);
Q_12 = Q(:,:,12);

kPx_vec = kP_file.kP(:,1);
kPy_vec = kP_file.kP(:,2);
kPz_vec = kP_file.kP(:,3);
kPphi_vec = kP_file.kP(:,4);
kPtheta_vec = kP_file.kP(:,5);
kPpsi_vec = kP_file.kP(:,6);

kDx_vec = kD_file.kD(:,1);
kDy_vec = kD_file.kD(:,2);
kDz_vec = kD_file.kD(:,3);
kDphi_vec = kD_file.kD(:,4);
kDtheta_vec = kD_file.kD(:,5);
kDpsi_vec = kD_file.kD(:,6);


x_vec_next = [curPos;curLinVel];
omega_vec_next = [curOrientation;curOrientationDot];
if x_vec_next(1) < X_min(1)
    n_x1 = 1;
elseif x_vec_next(1) > X_max(1)
    n_x1 = 26;
else
    n_x1 = floor(((x_vec_next(1)/(X_max(1)-X_min(1)))*N))+1;
end
if x_vec_next(2) < X_min(2)
    n_y1 = 1;
elseif x_vec_next(2) > X_max(2)
    n_y1 = 26;
else
    n_y1 = floor(((x_vec_next(2)/(X_max(2)-X_min(2)))*N))+1;
end
if x_vec_next(3) < X_min(3)
    n_z1 = 1;
elseif x_vec_next(3) > X_max(3)
    n_z1 = 26;
else
    n_z1 = floor(((x_vec_next(3)/(X_max(3)-X_min(3)))*N))+1;
end
if x_vec_next(4) < X_dot_min(1)
    n_x_dot1 = 1;
elseif x_vec_next(4) > X_dot_max(1)
    n_x_dot1 = 26;
else
    n_x_dot1 = floor(((x_vec_next(4)/(X_dot_max(1)-X_dot_min(1)))*N))+1;
end
if x_vec_next(5) < X_dot_min(2)
    n_y_dot1 = 1;
elseif x_vec_next(5) > X_dot_max(2)
    n_y_dot1 = 26;
else
    n_y_dot1 = floor(((x_vec_next(5)/(X_dot_max(2)-X_dot_min(2)))*N))+1;
end
if x_vec_next(6) < X_dot_min(3)
    n_z_dot1 = 1;
elseif x_vec_next(6) > X_dot_max(3)
    n_z_dot1 = 26;
else
    n_z_dot1 = floor(((x_vec_next(6)/(X_dot_max(3)-X_dot_min(3)))*N))+1;
end


if omega_vec_next(1) < omega_min(1)
    n_phi1 = 1;
elseif omega_vec_next(1) > omega_max(1)
    n_phi1 = 26;
else
    n_phi1 = floor(abs(((omega_vec_next(1)/(omega_max(1)-omega_min(1)))*N)))+1;
end
if omega_vec_next(2) < omega_min(2)
    n_theta1 = 1;
elseif omega_vec_next(2) > omega_max(2)
    n_theta1 = 26;
else
    n_theta1 = floor(abs(((omega_vec_next(2)/(omega_max(2)-omega_min(2)))*N)))+1;
end
if omega_vec_next(3) < omega_min(3)
    n_psi1 = 1;
elseif omega_vec_next(3) > omega_max(3)
    n_psi1 = 26;
else
    n_psi1 = floor(abs(((omega_vec_next(3)/(omega_max(3)-omega_min(3)))*N)))+1;
end
if omega_vec_next(4) < omega_dot_min(1)
    n_phi_dot1 = 1;
elseif omega_vec_next(4) > omega_dot_max(1)
    n_phi_dot1 = 26;
else
    n_phi_dot1 = floor(abs(((omega_vec_next(4)/(omega_dot_max(1)-omega_dot_min(1)))*N)))+1;
end
if omega_vec_next(5) < omega_dot_min(2)
    n_theta_dot1 = 1;
elseif omega_vec_next(5) > omega_dot_max(2)
    n_theta_dot1 = 26;
else
    n_theta_dot1 = floor(abs(((omega_vec_next(5)/(omega_dot_max(2)-omega_dot_min(2)))*N)))+1;
end
if omega_vec_next(6) < omega_dot_min(3)
    n_psi_dot1 = 1;
elseif omega_vec_next(6) > omega_dot_max(3)
    n_psi_dot1 = 26;
else
    n_psi_dot1 = floor(abs(((omega_vec_next(6)/(omega_dot_max(3)-omega_dot_min(3)))*N)))+1;
end


[~,ind1] = max(Q_1(n_x1,:));
[~,ind2] = max(Q_2(n_y1,:));
[~,ind3] = max(Q_3(n_z1,:));
[~,ind4] = max(Q_4(n_phi1,:));
[~,ind5] = max(Q_5(n_theta1,:));
[~,ind6] = max(Q_6(n_psi1,:));
[~,ind7] = max(Q_7(n_x_dot1,:));
[~,ind8] = max(Q_8(n_y_dot1,:));
[~,ind9] = max(Q_9(n_z_dot1,:));
[~,ind10] = max(Q_10(n_phi_dot1,:));
[~,ind11] = max(Q_11(n_theta_dot1,:));
[~,ind12] = max(Q_12(n_psi_dot1,:));

kPx = kPx_vec(ind1);
kPy = kPy_vec(ind2);
kPz = kPz_vec(ind3);
kPphi = kPphi_vec(ind4);
kPtheta = kPtheta_vec(ind5);
kPpsi = kPpsi_vec(ind6);

kDx = kDx_vec(ind7);
kDy = kDy_vec(ind8);
kDz = kDz_vec(ind9);
kDphi = kDphi_vec(ind10);
kDtheta = kDtheta_vec(ind11);
kDpsi = kDpsi_vec(ind12);
%
gain = [kPx;kPy;kPz;kPphi;kPtheta;kPpsi;kDx;kDy;kDz;kDphi;kDtheta;kDpsi];
end
